simulink model "actual_operation"  (R2022b)
settings: Solver=VariableStepAuto  StartTime=0.0  StopTime=5  RelTol=1e-3
values from neighbouring files (symbols this model uses):
  A = [ 0 1  0   0 ... (first row only)    [pole_config.m]
  A1 = A-B*k    [pole_config.m]
  B = [0 1 0 3]'    [pole_config.m]
  C = [ 1 0 0 0 ... (first row only)    [pole_config.m]
  D = [0 0]'    [pole_config.m]
settings Model: Creator=Administrator  LastModifiedBy=Rov
settings SolverCC: AlgebraicLoopSolver=TrustRegion
settings DataIOCC: ReturnWorkspaceOutputs=off
settings DebuggingCC: UnconnectedInputMsg=warning  UnconnectedOutputMsg=warning  UnconnectedLineMsg=warning  SFMachineParentedDataDiag=warning  ArithmeticOperatorsInVariantConditions=warning
settings ModelReferenceCC: EnableRefExpFcnMdlSchedulingChecks=on
settings SFSimCC: CustomCodeUndefinedFunction=UseInterfaceOnly

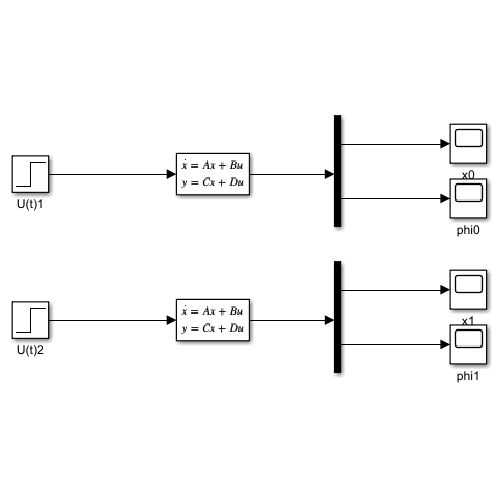
[thumbnail: Simulink's stored preview of the top-level diagram]
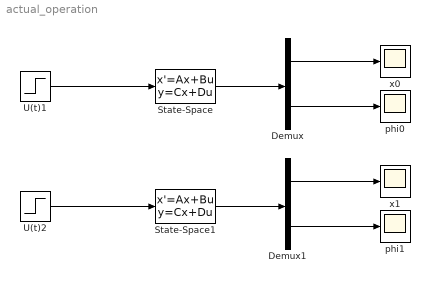
== system actual_operation ==
  Demux : Demux  Outputs=2
  Demux1 : Demux  Outputs=2
  State-Space : StateSpace  A=A  B=B  C=C  D=D  InitialCondition=0
  State-Space1 : StateSpace  A=A1  B=B  C=C  D=D  InitialCondition=0
  U(t)1 : Step  SampleTime=0
  U(t)2 : Step  SampleTime=0
  phi0 : Scope
  phi1 : Scope
  x0 : Scope
  x1 : Scope
  wires:
  State-Space/1 -> Demux/1
  U(t)1/1 -> State-Space/1
  U(t)2/1 -> State-Space1/1
  State-Space1/1 -> Demux1/1
  Demux/1 -> x0/1
  Demux/2 -> phi0/1
  Demux1/1 -> x1/1
  Demux1/2 -> phi1/1
